simulink model "distancetest"  (R2013a)
settings: Solver=ode3  SolverMode=SingleTasking  StartTime=0.0  StopTime=inf  RelTol=1e-3
values from neighbouring files (symbols this model uses):
  xf = cellfun(@str2num,txt2)    [interface.m]
undefined symbols (not defined in the file or in its folder): accel, handbrake, L, phi_lim, vlim, x0
libraries: legonxtlib x2
settings Model: SimulationMode=external  ExtModeTrigDuration=2  Creator=anton  LastModifiedBy=anton
settings OptimizationCC: OptimizeModelRefInitCode=on  LifeSpan=1
settings DebuggingCC: SolverPrmCheckMsg=none  StrictBusMsg=Warning
settings HardwareCC: ProdLargestAtomicInteger=Long  ProdLargestAtomicFloat=Float  ProdEndianess=LittleEndian  ProdHWDeviceType=ARM Compatible->ARM 7
settings RTWCC: SystemTargetFile=realtime.tlc  GenerateMakefile=off  TemplateMakefile=realtime.tmf  Description=Run on Target Hardware  RTWVerbose=off  ProcessScript=realtime_make_rtw_hook
settings STFCustomTargetCC: TargetLibSuffix=.a  GenerateSampleERTMain=on  ERTCustomFileBanners=on  SupportNonInlinedSFcns=off  SupportVariableSizeSignals=on  MATLABClassNameForMDSCustomization=Simulink.SoftwareTarget.ERTCustomization  SystemTargetFile=realtime.tlc
settings ERTTargetCC: ParMdlRefBuildCompliant=off  CompOptLevelCompliant=off  ConcurrentExecutionCompliant=off  CombineOutputUpdateFcns=off  ERTFirstTimeCompliant=off  SupportContinuousTime=on  SupportVariableSizeSignals=on  ModelStepFunctionPrototypeControlCompliant=off  CPPClassGenCompliant=off  ExtMode=on  ExtModeTransport=2  ExtModeMexFile=ext_serial_win32_comm_no_acks_rtt  ExtModeMexArgs=0 5 9600  ERTSrcFileBannerTemplate=realtime_code_template.cgt  ERTHdrFileBannerTemplate=realtime_code_template.cgt  ERTDataSrcFileTemplate=realtime_code_template.cgt  ERTDataHdrFileTemplate=realtime_code_template.cgt  ERTCustomFileTemplate=realtime_file_process.tlc

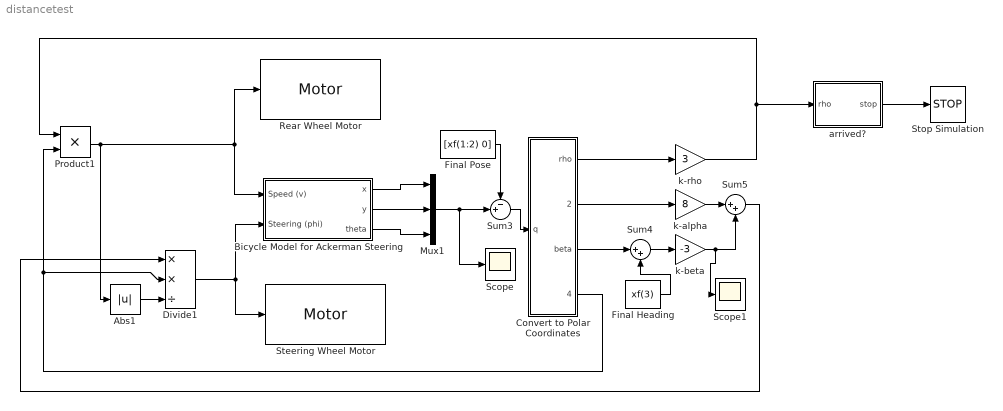
== system distancetest ==
  Abs1 : Abs
  Bicycle Model for Ackerman Steering : Subsystem
  Convert to Polar Coordinates : MATLAB Function  TreatAsAtomicUnit=on
  Divide1 : Product  Inputs=**/
  Final Heading : Constant  Value=xf(3)
  Final Pose : Constant  Value=[xf(1:2) 0]
  Mux1 : Mux  Inputs=3
  Product1 : Product  RndMeth=Zero
  Rear Wheel Motor : legonxtlib/Motor  sportNumber=C  sstopAction=Brake
  Scope : Scope
      settings: YMin=-2  YMax=15
  Scope1 : Scope
      settings: YMin=-2  YMax=15
  Steering Wheel Motor : legonxtlib/Motor  sportNumber=A  sstopAction=Brake
  Stop Simulation : Stop
  Sum3 : Sum  Inputs=-+|
  Sum4 : Sum  Inputs=|++
  Sum5 : Sum  Inputs=|++
  arrived? : MATLAB Function  TreatAsAtomicUnit=on
  k-alpha : Gain  Gain=8
  k-beta : Gain  Gain=-3
  k-rho : Gain  Gain=3
  wires:
  Bicycle Model for Ackerman Steering/2(y) -> Mux1/2
  Bicycle Model for Ackerman Steering/1(x) -> Mux1/1
  Bicycle Model for Ackerman Steering/3(theta) -> Mux1/3
  Mux1/1 -> Scope/1, Sum3/2
  Final Pose/1 -> Sum3/1
  Sum3/1 -> Convert to Polar Coordinates/1(q)
  Sum4/1 -> k-beta/1
  Convert to Polar Coordinates/3(beta) -> Sum4/1
  Final Heading/1 -> Sum4/2
  Abs1/1 -> Divide1/3
  Divide1/1 -> Steering Wheel Motor/1, Bicycle Model for Ackerman Steering/2(Steering (phi))
  k-alpha/1 -> Sum5/1
  k-beta/1 -> Scope1/1, Sum5/2
  Sum5/1 -> Divide1/1
  k-rho/1 -> Product1/1, arrived?/1(rho)
  Product1/1 -> Abs1/1, Rear Wheel Motor/1, Bicycle Model for Ackerman Steering/1(Speed (v))
  Convert to Polar Coordinates/4(direction) -> Product1/2, Divide1/2
  Convert to Polar Coordinates/2(alpha) -> k-alpha/1
  Convert to Polar Coordinates/1(rho) -> k-rho/1
  arrived?/1(stop) -> Stop Simulation/1

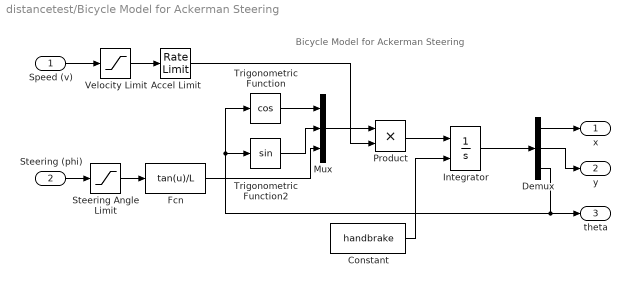
== system distancetest/Bicycle Model for Ackerman Steering ==
  note: Bicycle Model for Ackerman Steering
  Speed (v) : Inport
  Steering (phi) : Inport  Port=2
  Accel Limit : RateLimiter  RisingSlewLimit=accel  FallingSlewLimit=-accel  SampleTimeMode=inherited
  Constant : Constant  Value=handbrake
  Demux : Demux  Outputs=3
  Fcn : Fcn  Expr=tan(u)/L
  Integrator : Integrator  ExternalReset=level  InitialCondition=x0
  Mux : Mux  Inputs=3
  Product : Product  RndMeth=Zero
  Steering Angle Limit : Saturate  UpperLimit=phi_lim  LowerLimit=-phi_lim
  Trigonometric Function : Trigonometry  Operator=cos
  Trigonometric Function2 : Trigonometry
  Velocity Limit : Saturate  UpperLimit=vlim  LowerLimit=-vlim
  x : Outport
  y : Outport  Port=2
  theta : Outport  Port=3
  wires:
  Fcn/1 -> Mux/3
  Trigonometric Function/1 -> Mux/1
  Accel Limit/1 -> Product/2
  Product/1 -> Integrator/1
  Integrator/1 -> Demux/1
  Demux/3 -> Trigonometric Function/1, Trigonometric Function2/1, theta/1
  Demux/1 -> x/1
  Demux/2 -> y/1
  Steering (phi)/1 -> Steering Angle Limit/1
  Speed (v)/1 -> Velocity Limit/1
  Mux/1 -> Product/1
  Velocity Limit/1 -> Accel Limit/1
  Trigonometric Function2/1 -> Mux/2
  Steering Angle Limit/1 -> Fcn/1
  Constant/1 -> Integrator/2

== matlab function distancetest/arrived? ==
  data: rho input; stop output
function stop  = fcn(rho)  
    
    stop = 0;
    if double(abs(rho) < 0.08)
        stop = 1;
    end

== matlab function distancetest/Convert to Polar Coordinates ==
  data: q input; rho output; alpha output; beta output; direction output
function [rho, alpha, beta, direction] = fcn(q)  
    
    x = q(1); y = q(2); theta = q(3);

    rho = sqrt(x^2 + y^2);    % goal vector magnitude
    beta = -atan2(-y, -x);    % goal vector w.r.t. world frame
    alpha = -theta - beta;    % goal vector w.r.t. vehicle frame
    direction = 1;            % drive forward always
    
    
%     direction = 0;
%     % if first time in... 
%     if direction == 0
%         beta = -atan2(-y, -x);    % goal vector w.r.t. world frame
%         alpha = -theta - beta;    % goal vector w.r.t. vehicle frame
%         
%         % first time in simulation, choose the direction of travel
%         if (alpha > pi/2) || (alpha < -pi/2)
%             % fprintf('going backwards\n');
%             direction = -1;
%         else
%             % fprintf('going forwards\n');
%             direction = 1;
%         end
%     elseif direction == -1
%         beta = -atan2(y, x);
%         alpha = -theta - beta;
%     else
%         beta = -atan2(-y, -x);
%         alpha = -theta - beta;
%     end
%     
%     % cap alpha at +/- pi/2
%     if alpha > pi/2
%         alpha = pi/2;
%     end
%     if alpha < -pi/2
%         alpha = -pi/2;
%     end
